simulink model "Optimisation01"  (R2020b)
settings: Solver=FixedStepAuto  StartTime=0.0  StopTime=10  FixedStep=0.01  MaxStep=0.2  RelTol=1e-3
model workspace (MAT data in the model file):
  Optimisation01_sdosession = sldodialogs.data.SessionData
  Optimisation01_sdosession.Version = '3.0'
  Optimisation01_sdosession.Data.ModelName = 'Optimisation01'
  Optimisation01_sdosession.Data.ToolType = 'ResponseOptimization'
  Optimisation01_sdosession.Data.GUIOptions.NoPromptClose = 0
  Optimisation01_sdosession.Data.Workspace.LocalWorkspace.DesignVars(1) = param.Continuous
  Optimisation01_sdosession.Data.Workspace.LocalWorkspace.DesignVars(1).Scale_ = 128
  Optimisation01_sdosession.Data.Workspace.LocalWorkspace.DesignVars(1).Size_ = [1 1]
  Optimisation01_sdosession.Data.Workspace.LocalWorkspace.DesignVars(1).Value_ = 50.1084192258
  Optimisation01_sdosession.Data.Workspace.LocalWorkspace.DesignVars(1).pID = paramid.Variable
  Optimisation01_sdosession.Data.Workspace.LocalWorkspace.DesignVars(1).pID.Name = 'Kd'
  Optimisation01_sdosession.Data.Workspace.LocalWorkspace.DesignVars(2) = param.Continuous
  Optimisation01_sdosession.Data.Workspace.LocalWorkspace.DesignVars(2).Scale_ = 8
  Optimisation01_sdosession.Data.Workspace.LocalWorkspace.DesignVars(2).Size_ = [1 1]
  Optimisation01_sdosession.Data.Workspace.LocalWorkspace.DesignVars(2).Value_ = 6.29568850936
  Optimisation01_sdosession.Data.Workspace.LocalWorkspace.DesignVars(2).pID = paramid.Variable
  Optimisation01_sdosession.Data.Workspace.LocalWorkspace.DesignVars(2).pID.Name = 'Ki'
  Optimisation01_sdosession.Data.Workspace.LocalWorkspace.DesignVars(3) = param.Continuous
  Optimisation01_sdosession.Data.Workspace.LocalWorkspace.DesignVars(3).Scale_ = 512
  Optimisation01_sdosession.Data.Workspace.LocalWorkspace.DesignVars(3).Size_ = [1 1]
  Optimisation01_sdosession.Data.Workspace.LocalWorkspace.DesignVars(3).Value_ = 364.260452278
  Optimisation01_sdosession.Data.Workspace.LocalWorkspace.DesignVars(3).pID = paramid.Variable
  Optimisation01_sdosession.Data.Workspace.LocalWorkspace.DesignVars(3).pID.Name = 'Kp'
  Optimisation01_sdosession.Data.Workspace.LocalWorkspace.ReqValues.Name = 'SignalProperty'
  Optimisation01_sdosession.Data.Workspace.LocalWorkspace.ReqValues.Type = 'min'
  Optimisation01_sdosession.Data.Workspace.LocalWorkspace.ReqValues.Value = 0.138601422932
  Optimisation01_sdosession.Data.Workspace.LocalWorkspace.ReqValues.DisplayValue = 0.138601422932
  Optimisation01_sdosession.Data.Workspace.LocalWorkspace.ReqValues_1.Name = 'SignalProperty'
  Optimisation01_sdosession.Data.Workspace.LocalWorkspace.ReqValues_1.Type = 'min'
  Optimisation01_sdosession.Data.Workspace.LocalWorkspace.ReqValues_1.Value = 0.264162161638
  Optimisation01_sdosession.Data.Workspace.LocalWorkspace.ReqValues_1.DisplayValue = 0.264162161638
  Optimisation01_sdosession.Data.Workspace.LocalWorkspace.Sig = Simulink.SimulationData.Signal
  Optimisation01_sdosession.Data.Workspace.LocalWorkspace.Sig.PortType = 'outport'
  Optimisation01_sdosession.Data.Workspace.LocalWorkspace.Sig.Version = 1
  Optimisation01_sdosession.Data.Workspace.LocalWorkspace.Sig.BlockPath = Simulink.SimulationData.BlockPath
  Optimisation01_sdosession.Data.Workspace.LocalWorkspace.Sig.BlockPath.path = {'Optimisation01/Sqrt'}
  Optimisation01_sdosession.Data.Workspace.LocalWorkspace.SignalProperty = sdo.requirements.SignalProperty
  Optimisation01_sdosession.Data.Workspace.LocalWorkspace.SignalProperty.sdo.requirements.Requirement.Data_ : srorequirement.functiondata (value not decoded)
  Optimisation01_sdosession.Data.Workspace.LocalWorkspace.SignalProperty.sdo.requirements.Requirement.Check_ = sdo.requirements.ScalarCheck
  Optimisation01_sdosession.Data.Workspace.HiddenWorkspace = []
  Optimisation01_sdosession.Data.ToolData.PlotManager.Plots(1).Class = 'sldoplots.TimePlot'
  Optimisation01_sdosession.Data.ToolData.PlotManager.Plots(1).Sources = {'Sig'}
  Optimisation01_sdosession.Data.ToolData.PlotManager.Plots(2).Class = 'sldoplots.IterPlot'
  Optimisation01_sdosession.Data.ToolData.PlotManager.Plots(2).Sources = {'SignalProperty'}
  Optimisation01_sdosession.Data.ToolData.PlotManager.Tiling : java.lang.String (value not decoded)
  Optimisation01_sdosession.Data.ToolData.DialogManager = []
  Optimisation01_sdosession.Data.ToolData.ResponseOptimization.Options = sdo.OptimizeOptions
  Optimisation01_sdosession.Data.ToolData.ResponseOptimization.Options.OptimizedModel = 'Optimisation01'
  Optimisation01_sdosession.Data.ToolData.ResponseOptimization.Options.Version = 2
  Optimisation01_sdosession.Data.ToolData.ResponseOptimization.GUIOptions.ModelTimeOut = Inf
  Optimisation01_sdosession.Data.ToolData.ResponseOptimization.GUIOptions.ComputeOperatingPoint = 0
  Optimisation01_sdosession.Data.ToolData.ResponseOptimization.GUIOptions.ShowProgress = 1
  Optimisation01_sdosession.Data.ToolData.ResponseOptimization.GUIOptions.ShowParamTrajectory = 1
  Optimisation01_sdosession.Data.ToolData.ResponseOptimization.GUIOptions.UpdatePlots = 1
  Optimisation01_sdosession.Data.ToolData.ResponseOptimization.GUIOptions.UpdateModel = 1
  Optimisation01_sdosession.Data.ToolData.ResponseOptimization.GUIOptions.UpdateDesign = 'overwrite'
  Optimisation01_sdosession.Data.ToolData.ResponseOptimization.GUIOptions.SaveReport = 0
  Optimisation01_sdosession.Data.ToolData.ResponseOptimization.GUIOptions.SaveRequirementValue = 1
  Optimisation01_sdosession.Data.ToolData.ResponseOptimization.LinOptions = linearize.LinearizeOptions
  Optimisation01_sdosession.Data.ToolData.ResponseOptimization.RequirementOperatingPointSetup = []
  Optimisation01_sdosession.Data.ToolData.ResponseOptimization.LocalRequirements.Requirement = 'SignalProperty'
  Optimisation01_sdosession.Data.ToolData.ResponseOptimization.LocalRequirements.Source = {'Sig'}
  Optimisation01_sdosession.Data.ToolData.ResponseOptimization.LocalRequirements.Selected = 1
  Optimisation01_sdosession.Data.ToolData.ResponseOptimization.BlockRequirements = struct([])
  Optimisation01_sdosession.Data.ToolData.ResponseOptimization.LocalExperiments = struct([])
  Optimisation01_sdosession.Data.ToolData.ResponseOptimization.Cost.Type = 'SSE'
  Optimisation01_sdosession.Data.ToolData.ResponseOptimization.Cost.Robust = 'off'
  Optimisation01_sdosession.Data.ToolData.ResponseOptimization.DesignVariables = 'DesignVars'
  Optimisation01_sdosession.Data.ToolData.ResponseOptimization.UncertainVariables = ''
  Optimisation01_sdosession.Data.ToolData.ResponseOptimization.DataToPlot = 'Sig'
values from neighbouring files (symbols this model uses):
  Kd = 138.349198174    [OptimisationData.mat]    (also in myCustomRequirement.m = data.DesignVars(3))
  Ki = 3.37771766611    [OptimisationData.mat]    (also in myCustomRequirement.m = data.DesignVars(2))
  Kp = 1303.85880325    [OptimisationData.mat]    (also in myCustomRequirement.m = data.DesignVars(1))
  Power = [0 0.135039524161 8.91914965689 7.78138466797 9.0073673393 8.96604203154 8.86759000228 15.68308669 17.9316117445 18.8693109472 25.7680840998 34.2690025221 ... (50 elements, 50x1)]    [MotorData.mat]    (also in OptimisationData.mat = [0 0.134792669981 8.9180951627 7.77881648635 9.00749423422 8)
  Throttle = [0 1 2.66666666667 3.44444444444 6.55555555556 8.11111111111 8.88888888889 13.6666666667 14.4444444444 15.2222222222 18.3333333333 21.5555555556 ... (50 elements, 50x1)]    [MotorData.mat]    (also in OptimisationData.mat)
  Thrust = [0 0.00386703849483 0.447248955951 0.381725752671 0.429816366755 0.448130327307 0.434268732353 0.786362880096 0.850043356053 0.907127881895 1.24377109743 1.5194958901 ... (50 elements, 50x1)]    [MotorData.mat]    (also in OptimisationData.mat)
libraries: simulink x2, pid_lib x1
settings Model: Creator=IR13  LastModifiedBy=IR13
settings SolverCC: ZeroCrossAlgorithm=Adaptive
settings DataIOCC: Refine=2
settings OptimizationCC: DefaultUnderspecifiedDataType=single
settings DebuggingCC: IgnoredZcDiagnostic=none

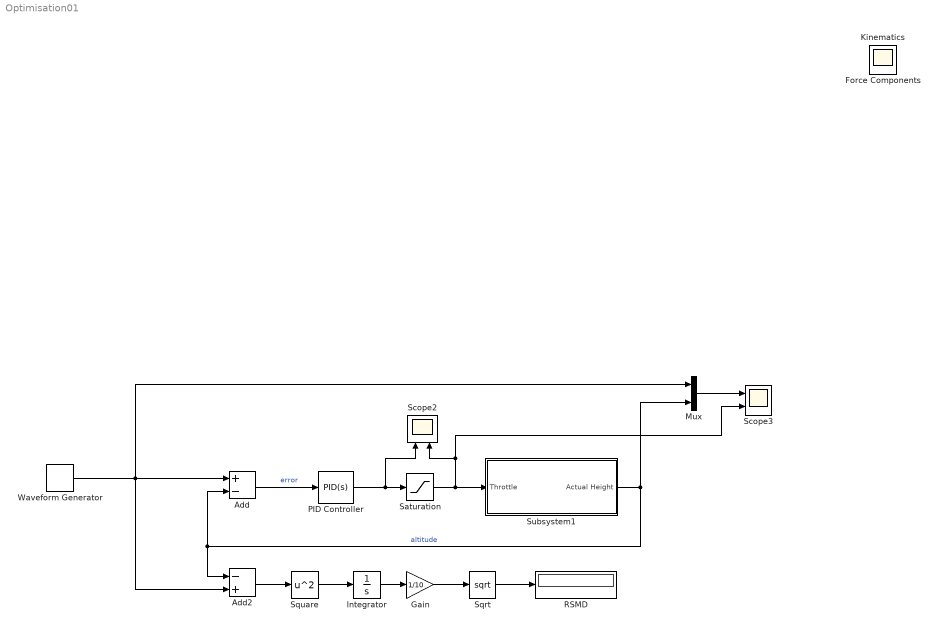
== system Optimisation01 ==
  Add : Sum  Inputs=+-
  Add2 : Sum  Inputs=-+
  Gain : Gain  Gain=1/10
  Integrator : Integrator
  Mux : Mux  Inputs=2
  PID Controller : pid_lib/PID Controller  Controller=PID  Form=Parallel  TimeDomain=Continuous-time  UseExternalTs=off  SampleTime=-1  IntegratorMethod=Forward Euler  FilterMethod=Forward Euler  ControllerParametersSource=internal  P=Kp  I=Ki  D=Kd  UseFilter=on  N=100  TunerSelectOption=Transfer Function Based (PID Tuner App)  InitialConditionSource=internal  InitialConditionForIntegrator=0  InitialConditionForFilter=0  DifferentiatorICPrevScaledInput=0  ExternalReset=none  TrackingMode=off  Kt=1  LimitOutput=off  SatLimitsSource=internal  UpperSaturationLimit=inf  LowerSaturationLimit=-inf  LinearizeAsGain=on  AntiWindupMode=none  Kb=1  POutMin=[]  POutMax=[]  IOutMin=[]  IOutMax=[]  DOutMin=[]  DOutMax=[]  NOutMin=[]  NOutMax=[]  SumOutMin=[]  SumOutMax=[]  SaturationOutMin=[]  SaturationOutMax=[]  PParamMin=[]  PParamMax=[]  IParamMin=[]  IParamMax=[]  DParamMin=[]  DParamMax=[]  NParamMin=[]  NParamMax=[]  KbParamMin=[]  KbParamMax=[]  KtParamMin=[]  KtParamMax=[]  KbOutMin=[]  KbOutMax=[]  KtOutMin=[]  KtOutMax=[]  IntegratorOutMin=[]  IntegratorOutMax=[]  FilterOutMin=[]  FilterOutMax=[]  SumI1OutMin=[]  SumI1OutMax=[]  SumI2OutMin=[]  SumI2OutMax=[]  SumI3OutMin=[]  SumI3OutMax=[]  SumI4OutMin=[]  SumI4OutMax=[]  SumDOutMin=[]  SumDOutMax=[]  DifferentiatorOutMin=[]  DifferentiatorOutMax=[]  FilterDiffOutCoefMin=[]  FilterDiffOutCoefMax=[]  ReciprocalOutMin=[]  ReciprocalOutMax=[]  SumDenOutMin=[]  SumDenOutMax=[]  SumNumOutMin=[]  SumNumOutMax=[]  DivideOutMin=[]  DivideOutMax=[]  UdiffTsProdOutMin=[]  UdiffTsProdOutMax=[]  NTsProdOutMin=[]  NTsProdOutMax=[]  UintegralTsProdOutMin=[]  UintegralTsProdOutMax=[]  UngainTsProdOutMin=[]  UngainTsProdOutMax=[]  IntegratorContinuousStateAttributes=''  IntegratorStateMustResolveToSignalObject=off  IntegratorRTWStateStorageClass=Auto  FilterContinuousStateAttributes=''  FilterStateMustResolveToSignalObject=off  FilterRTWStateStorageClass=Auto  ParallelPVariant=InternalParameters  IdealPVariant=Disabled  IVariant=InternalParameters  DVariant=InternalParameters  IntegratorVariant=Continuous  SatVariant=Disabled  AWVariant=Passthrough  PCopyVariant=Disabled  TRVariant=Disabled  FdbkBlocksVariant=Forward  IdealPFdbkVariant=Disabled  SatFdbkVariant=Disabled  DerivativeFilterVariant=ContFilter  NVariant=InternalParameters  NCopyVariant=Disabled  FilterICVariant=InternalICsFilter  IntegratorICVariant=InternalICs  ExternalResetVariant=Disabled  TRSumVariant=Passthrough  SumFdbkVariant=Disabled  SumVariant=Sum_PID  TsampFilterVariant=InternalTs  TsampNgainVariant=Passthrough  TsampIntegralVariant=Passthrough  ExternalSaturationOutDataTypeStr=Inherit: Same as second input
  RSMD : Display
  Saturation : Saturate  UpperLimit=100  LowerLimit=0
  Scope2 : Scope  NumInputPorts=2
  Scope3 : Scope  NumInputPorts=2
  Sqrt : Sqrt  SaturateOnIntegerOverflow=on
  Square : Math  Operator=square  SaturateOnIntegerOverflow=on
  Subsystem1 : Subsystem
  Waveform Generator : simulink/Sources/Waveform Generator  OutMin=[]  OutMax=[]  OutDataTypeStr=double  SelectedSignal=1  Signals=pulse(0.5, 2, 2) + pulse(1,5,2) + pulse(0.5,6,2)#pulse(1,4,2)#pulse(0.5,6,2)  BlockNames=MultiportSwitch_1f4ce5d91b3e4fe#MultiportSwitch_6a89107336d5467#MultiportSwitch_35f949fc017b494  SampleTime=0.1
  Force Components : Scope
  Kinematics : Scope
  wires:
  Saturation/1 -> Scope3/2, Scope2/2, Subsystem1/1(Throttle)
  Add2/1 -> Square/1
  Gain/1 -> Sqrt/1
  Add/1 -> PID Controller/1  "error"
  Waveform Generator/1 -> Mux/1, Add/1, Add2/2
  Square/1 -> Integrator/1
  Subsystem1/1(Actual Height) -> Mux/2, Add2/1, Add/2  "altitude"
  Sqrt/1 -> RSMD/1
  PID Controller/1 -> Scope2/1, Saturation/1
  Integrator/1 -> Gain/1
  Mux/1 -> Scope3/1

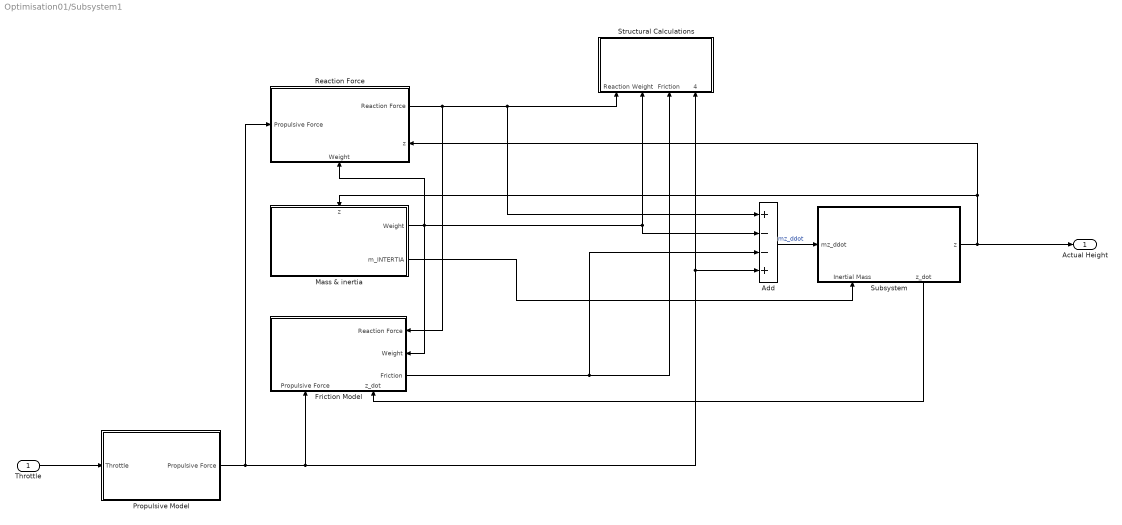
== system Optimisation01/Subsystem1 ==
  Throttle : Inport
  Add : Sum  Inputs=+--+
  Friction Model : Subsystem
      settings: PortSchema="{\"entries\":[{\"content\":{\"sides\":[{\"content\":{\"connectorIds\":[]},\"type\":\"ConnectorPlacement.EquallySpacedRectSide\",\"uuid\":\"1b3e095a-62ff-489c-96d9-63a8a1a842c7\"},{\"content\":{\"connectorIds\":[\"In3\",\"In4\",\"Out1\"],\"side\":\"RIGHT\"},\"type\":\"ConnectorPlacement.EquallySpacedRectSide\",\"uuid\":\"2aa3988f-f37b-48ca-a763-ece382c29199\"},{\"content\":{\"connectorIds\":[],\"side\":\"TOP\"},\"type\":\"ConnectorPlacement.EquallySpacedRectSide\",\"uuid\":\"ef7ffbd1-84d2-4291-ae41-90f24840b975\"},{\"content\":{\"connectorIds\":[\"In1\",\"In2\"],\"side\":\"BOTTOM\"},\"type\":\"ConnectorPlacement.EquallySpacedRectSide\",\"uuid\":\"ca187e87-455c-44d4-b2d5-496c3fe29e76\"},{\"content\":{\"connectorIds\":[],\"side\":\"HIDDEN\"},\"type\":\"ConnectorPlacement.EquallySpacedRectSide\",\"uuid\":\"11859c76-ab54-4977-b256-12d02241e5aa\"}]},\"type\":\"ConnectorPlacement.EquallySpacedConnector\",\"uuid\":\"162037a6-f725-4d16-a5f0-9112b8e8c48a\"}],\"packageUris\":[\"http://schema.mathworks.com/mf0/Connector/R2020b\"],\"version\":\"1.0\"}"
  Mass & inertia : Subsystem
      settings: PortSchema="{\"entries\":[{\"content\":{\"sides\":[{\"content\":{\"connectorIds\":[]},\"type\":\"ConnectorPlacement.EquallySpacedRectSide\",\"uuid\":\"1399d11e-8fed-4a75-a6ac-2b525e4dbe81\"},{\"content\":{\"connectorIds\":[\"Out1\",\"Out2\"],\"side\":\"RIGHT\"},\"type\":\"ConnectorPlacement.EquallySpacedRectSide\",\"uuid\":\"2e2e7a23-dcb2-4001-96a5-c1562d5723c6\"},{\"content\":{\"connectorIds\":[\"In1\"],\"side\":\"TOP\"},\"type\":\"ConnectorPlacement.EquallySpacedRectSide\",\"uuid\":\"b0373260-5e1a-43dd-bca8-24421c20e285\"},{\"content\":{\"connectorIds\":[],\"side\":\"HIDDEN\"},\"type\":\"ConnectorPlacement.EquallySpacedRectSide\",\"uuid\":\"35e9db29-fffd-4860-9f0e-8f51711f4d01\"}]},\"type\":\"ConnectorPlacement.EquallySpacedConnector\",\"uuid\":\"39bd9006-0e99-41e8-8a89-05408a55c646\"}],\"packageUris\":[\"http://schema.mathworks.com/mf0/Connector/R2020b\"],\"version\":\"1.0\"}"
  Propulsive Model : Subsystem
  Reaction Force : Subsystem
      settings: PortSchema="{\"entries\":[{\"content\":{\"sides\":[{\"content\":{\"connectorIds\":[\"In1\"]},\"type\":\"ConnectorPlacement.EquallySpacedRectSide\",\"uuid\":\"1e35d603-08eb-402b-a2de-16d799202cf1\"},{\"content\":{\"connectorIds\":[\"Out1\",\"In3\"],\"side\":\"RIGHT\"},\"type\":\"ConnectorPlacement.EquallySpacedRectSide\",\"uuid\":\"6309f8f8-5c50-477a-b178-9a414ecebc78\"},{\"content\":{\"connectorIds\":[],\"side\":\"TOP\"},\"type\":\"ConnectorPlacement.EquallySpacedRectSide\",\"uuid\":\"1075b443-bbcc-4bf5-9b05-7b44ecc9bacc\"},{\"content\":{\"connectorIds\":[\"In2\"],\"side\":\"BOTTOM\"},\"type\":\"ConnectorPlacement.EquallySpacedRectSide\",\"uuid\":\"9465d0d7-9803-4a37-84cd-7fa866de481e\"},{\"content\":{\"connectorIds\":[],\"side\":\"HIDDEN\"},\"type\":\"ConnectorPlacement.EquallySpacedRectSide\",\"uuid\":\"80b90c9b-51c1-4183-87d9-243ed5e6c391\"}]},\"type\":\"ConnectorPlacement.EquallySpacedConnector\",\"uuid\":\"514452d4-5b8b-4aa9-8f6a-f7d3b564ce33\"}],\"packageUris\":[\"http://schema.mathworks.com/mf0/Connector/R2020b\"],\"version\":\"1.0\"}"
  Structural Calculations : Subsystem
  Subsystem : Subsystem
      settings: PortSchema="{\"entries\":[{\"content\":{\"sides\":[{\"content\":{\"connectorIds\":[\"In1\"]},\"type\":\"ConnectorPlacement.EquallySpacedRectSide\",\"uuid\":\"4280b032-842d-4d16-b8c5-b63b72592cbb\"},{\"content\":{\"connectorIds\":[\"Out1\"],\"side\":\"RIGHT\"},\"type\":\"ConnectorPlacement.EquallySpacedRectSide\",\"uuid\":\"e4e0b7b9-12b8-4ae8-8e3c-cb8798002b22\"},{\"content\":{\"connectorIds\":[],\"side\":\"TOP\"},\"type\":\"ConnectorPlacement.EquallySpacedRectSide\",\"uuid\":\"d9ed1db6-3da5-4dd5-916f-0a0888e518e7\"},{\"content\":{\"connectorIds\":[\"In2\",\"Out2\"],\"side\":\"BOTTOM\"},\"type\":\"ConnectorPlacement.EquallySpacedRectSide\",\"uuid\":\"d18e58c7-4d86-4b90-a916-d0a361083c2d\"},{\"content\":{\"connectorIds\":[],\"side\":\"HIDDEN\"},\"type\":\"ConnectorPlacement.EquallySpacedRectSide\",\"uuid\":\"56aebb37-ad12-4a95-93b1-0a5b21e6f2e4\"}]},\"type\":\"ConnectorPlacement.EquallySpacedConnector\",\"uuid\":\"f0e8b7a0-91bd-4506-81db-435517f4e301\"}],\"packageUris\":[\"http://schema.mathworks.com/mf0/Connector/R2020b\"],\"version\":\"1.0\"}"
  Actual Height : Outport
  wires:
  Reaction Force/1(Reaction Force) -> Add/1, Structural Calculations/1(Reaction), Friction Model/3(Reaction Force)
  Mass & inertia/2(m_INTERTIA) -> Subsystem/2(Inertial Mass)
  Throttle/1 -> Propulsive Model/1(Throttle)
  Subsystem/1(z) -> Actual Height/1, Reaction Force/3(z), Mass & inertia/1(z)
  Subsystem/2(z_dot) -> Friction Model/2(z_dot)
  Propulsive Model/1(Propulsive Force) -> Add/4, Structural Calculations/4(Propulsion), Friction Model/1(Propulsive Force), Reaction Force/1(Propulsive Force)
  Add/1 -> Subsystem/1(mz_ddot)  "mz_ddot"
  Mass & inertia/1(Weight) -> Friction Model/4(Weight), Reaction Force/2(Weight), Structural Calculations/2(Weight), Add/2
  Friction Model/1(Friction) -> Add/3, Structural Calculations/3(Friction)

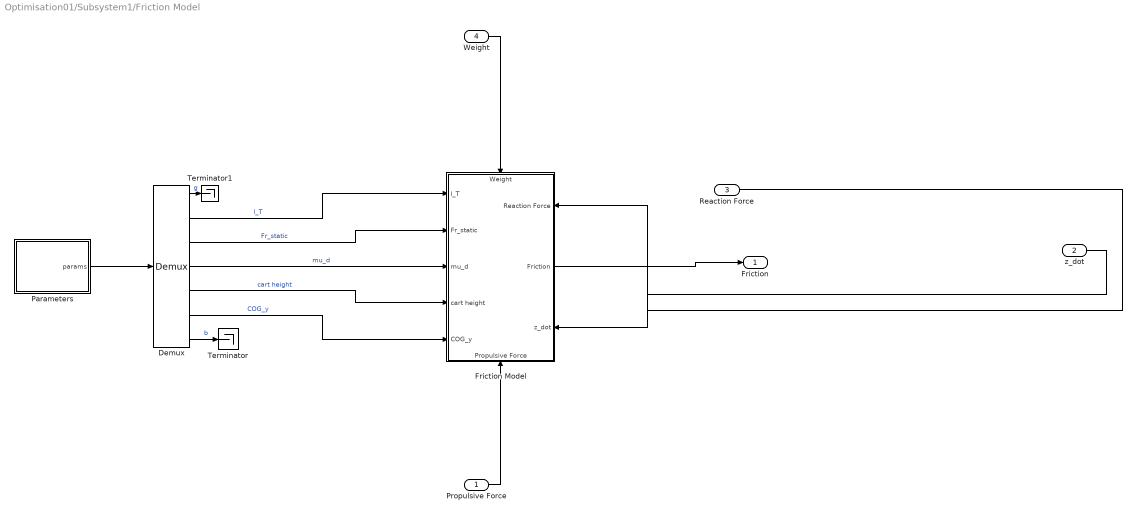
== system Optimisation01/Subsystem1/Friction Model ==
  Propulsive Force : Inport
  z_dot : Inport  Port=2
  Reaction Force : Inport  Port=3
  Weight : Inport  Port=4
  Demux : Demux  Outputs=7
  Friction Model : Subsystem
      settings: PortSchema="{\"entries\":[{\"content\":{\"sides\":[{\"content\":{\"connectorIds\":[\"In1\",\"In2\",\"In3\",\"In4\",\"In5\"]},\"type\":\"ConnectorPlacement.EquallySpacedRectSide\",\"uuid\":\"b80da770-fdb0-4d6f-bea5-94e06f2afa04\"},{\"content\":{\"connectorIds\":[\"In8\",\"Out1\",\"In9\"],\"side\":\"RIGHT\"},\"type\":\"ConnectorPlacement.EquallySpacedRectSide\",\"uuid\":\"44cc0c5b-7bc2-4d7d-ab9c-4e4237bff03f\"},{\"content\":{\"connectorIds\":[\"In6\"],\"side\":\"TOP\"},\"type\":\"ConnectorPlacement.EquallySpacedRectSide\",\"uuid\":\"d8cf9831-f5c9-4bfd-8650-bb94040859dc\"},{\"content\":{\"connectorIds\":[\"In7\"],\"side\":\"BOTTOM\"},\"type\":\"ConnectorPlacement.EquallySpacedRectSide\",\"uuid\":\"5dc8ad5a-b457-4b35-ae96-3ded03a76763\"},{\"content\":{\"connectorIds\":[],\"side\":\"HIDDEN\"},\"type\":\"ConnectorPlacement.EquallySpacedRectSide\",\"uuid\":\"8dab3da8-cd9e-407c-8850-bafd2d7a131e\"}]},\"type\":\"ConnectorPlacement.EquallySpacedConnector\",\"uuid\":\"d0f16782-5cb8-4cea-b1e1-f78879901c5f\"}],\"packageUris\":[\"http://schema.mathworks.com/mf0/Connector/R2020b\"],\"version\":\"1.0\"}"
  Parameters : MATLAB Function  TreatAsAtomicUnit=on
  Terminator : Terminator
  Terminator1 : Terminator
  Friction : Outport
  wires:
  Demux/7 -> Terminator/1  "b"
  Reaction Force/1 -> Friction Model/8(Reaction Force)
  Demux/1 -> Terminator1/1  "g"
  Propulsive Force/1 -> Friction Model/7(Propulsive Force)
  Demux/2 -> Friction Model/1(l_T)  "l_T"
  Friction Model/1(Friction) -> Friction/1
  Weight/1 -> Friction Model/6(Weight)
  Demux/3 -> Friction Model/2(Fr_static)  "Fr_static"
  Parameters/1(params) -> Demux/1
  Demux/4 -> Friction Model/3(mu_d)  "mu_d"
  z_dot/1 -> Friction Model/9(z_dot)
  Demux/5 -> Friction Model/4(cart height)  "cart height"
  Demux/6 -> Friction Model/5(COG_y)  "COG_y"

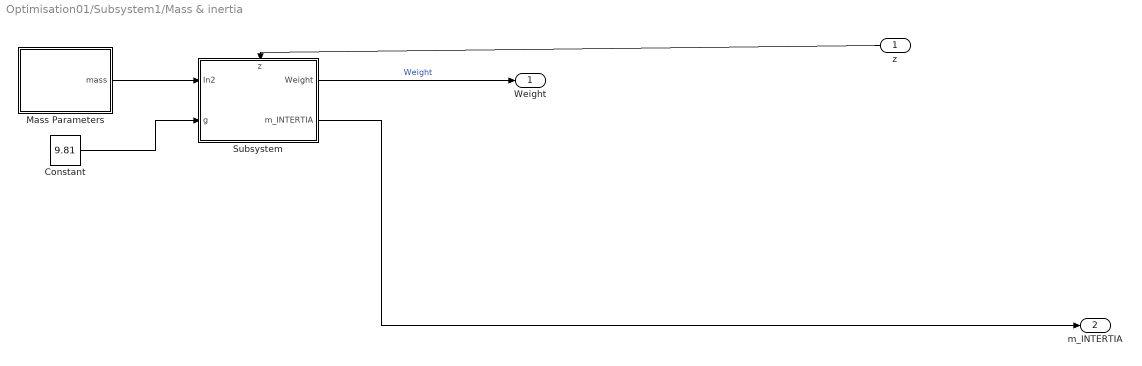
== system Optimisation01/Subsystem1/Mass & inertia ==
  z : Inport
  Constant : Constant  Value=9.81
  Mass Parameters : MATLAB Function  TreatAsAtomicUnit=on
  Subsystem : Subsystem
      settings: PortSchema="{\"entries\":[{\"content\":{\"sides\":[{\"content\":{\"connectorIds\":[\"In1\",\"In2\"]},\"type\":\"ConnectorPlacement.EquallySpacedRectSide\",\"uuid\":\"22ad1645-0c4a-4eab-a942-e35708909bc2\"},{\"content\":{\"connectorIds\":[\"Out1\",\"Out2\"],\"side\":\"RIGHT\"},\"type\":\"ConnectorPlacement.EquallySpacedRectSide\",\"uuid\":\"049dc02c-af21-4242-96fd-198a717a970b\"},{\"content\":{\"connectorIds\":[\"In3\"],\"side\":\"TOP\"},\"type\":\"ConnectorPlacement.EquallySpacedRectSide\",\"uuid\":\"a1727784-13c5-452f-b8c4-4da743b82409\"},{\"content\":{\"connectorIds\":[],\"side\":\"HIDDEN\"},\"type\":\"ConnectorPlacement.EquallySpacedRectSide\",\"uuid\":\"a08d060c-4763-496d-ac54-202c99d24543\"}]},\"type\":\"ConnectorPlacement.EquallySpacedConnector\",\"uuid\":\"dcd15304-2046-43f2-990d-e6438030fbb8\"}],\"packageUris\":[\"http://schema.mathworks.com/mf0/Connector/R2020b\"],\"version\":\"1.0\"}"
  Weight : Outport
  m_INTERTIA : Outport  Port=2
  wires:
  Subsystem/2(m_INTERTIA) -> m_INTERTIA/1
  Constant/1 -> Subsystem/2(g)
  Subsystem/1(Weight) -> Weight/1  "Weight"
  z/1 -> Subsystem/3(z)
  Mass Parameters/1(mass) -> Subsystem/1(In2)

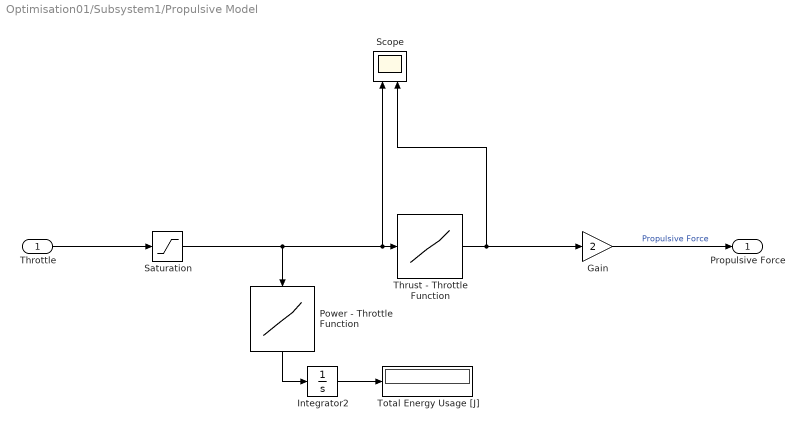
== system Optimisation01/Subsystem1/Propulsive Model ==
  Throttle : Inport
  Gain : Gain  Gain=2
  Integrator2 : Integrator
  Power - Throttle Function : Lookup_n-D  NumberOfTableDimensions=1  BreakpointsForDimension1=Throttle  BreakpointsForDimension2=[1:3]  Table=Power  ExtrapMethod=Clip  InternalRulePriority=Speed  RndMeth=Simplest  InputSameDT=on
  Saturation : Saturate  UpperLimit=100  LowerLimit=0
  Scope : Scope  NumInputPorts=2
  Thrust - Throttle Function : Lookup_n-D  NumberOfTableDimensions=1  BreakpointsForDimension1=Throttle  BreakpointsForDimension2=[1:3]  Table=Thrust  ExtrapMethod=Clip  DiagnosticForOutOfRangeInput=Warning  InternalRulePriority=Speed  RndMeth=Simplest  InputSameDT=on
  Total Energy Usage [J] : Display
  Propulsive Force : Outport
  wires:
  Integrator2/1 -> Total Energy Usage [J]/1
  Thrust - Throttle Function/1 -> Gain/1, Scope/2
  Power - Throttle Function/1 -> Integrator2/1
  Gain/1 -> Propulsive Force/1  "Propulsive Force"
  Throttle/1 -> Saturation/1
  Saturation/1 -> Scope/1, Thrust - Throttle Function/1, Power - Throttle Function/1

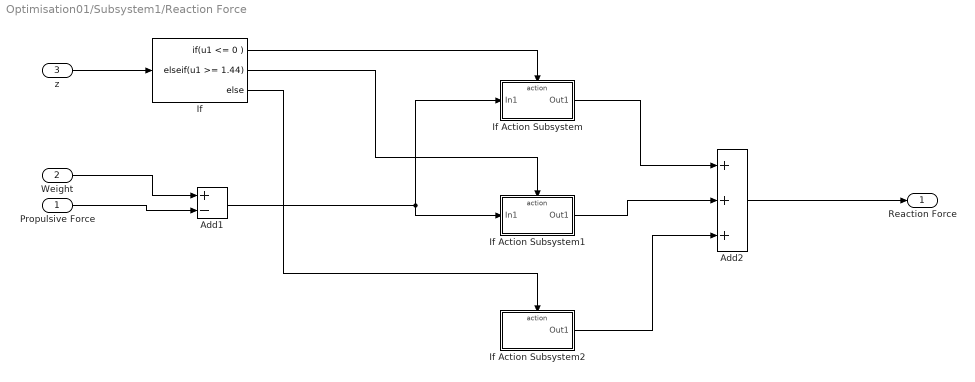
== system Optimisation01/Subsystem1/Reaction Force ==
  Propulsive Force : Inport
  Weight : Inport  Port=2
  z : Inport  Port=3
  Add1 : Sum  Inputs=+-
  Add2 : Sum  Inputs=+++
  If : If  IfExpression=u1 <= 0  ElseIfExpressions=u1 >= 1.44
  If Action Subsystem : Subsystem  TreatAsAtomicUnit=on
  If Action Subsystem1 : Subsystem  TreatAsAtomicUnit=on
  If Action Subsystem2 : Subsystem  TreatAsAtomicUnit=on
  Reaction Force : Outport
  wires:
  Weight/1 -> Add1/1
  If Action Subsystem1/1(Out1) -> Add2/2
  z/1 -> If/1
  Add2/1 -> Reaction Force/1
  If/2 -> If Action Subsystem1/Action
  If Action Subsystem2/1(Out1) -> Add2/3
  Propulsive Force/1 -> Add1/2
  If Action Subsystem/1(Out1) -> Add2/1
  If/3 -> If Action Subsystem2/Action
  If/1 -> If Action Subsystem/Action
  Add1/1 -> If Action Subsystem1/1(In1), If Action Subsystem/1(In1)

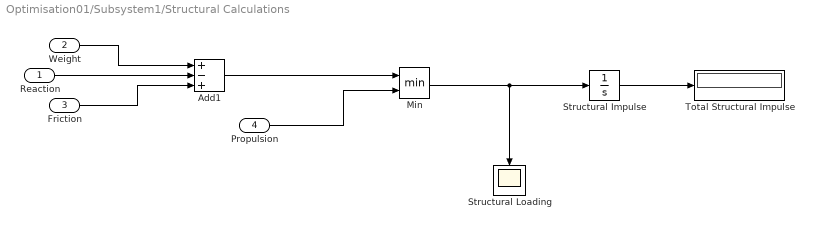
== system Optimisation01/Subsystem1/Structural Calculations ==
  Reaction : Inport
  Weight : Inport  Port=2
  Friction : Inport  Port=3
  Propulsion : Inport  Port=4
  Add1 : Sum  Inputs=+-+
  Min : MinMax  Inputs=2
  Structural Impulse : Integrator
  Structural Loading : Scope
  Total Structural Impulse : Display
  wires:
  Propulsion/1 -> Min/2
  Friction/1 -> Add1/3
  Min/1 -> Structural Loading/1, Structural Impulse/1
  Weight/1 -> Add1/1
  Reaction/1 -> Add1/2
  Structural Impulse/1 -> Total Structural Impulse/1
  Add1/1 -> Min/1

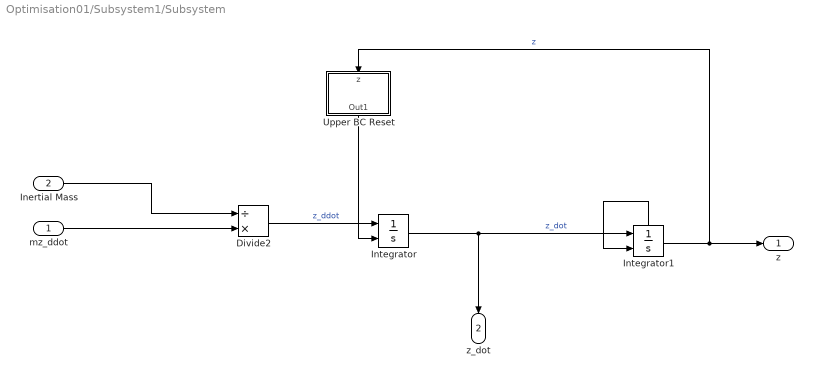
== system Optimisation01/Subsystem1/Subsystem ==
  mz_ddot : Inport
  Inertial Mass : Inport  Port=2
  Divide2 : Product  Inputs=/*
  Integrator : Integrator  ExternalReset=falling
  Integrator1 : Integrator  ExternalReset=falling  ShowStatePort=on
  Upper BC Reset : Subsystem
  z : Outport
  z_dot : Outport  Port=2
  wires:
  mz_ddot/1 -> Divide2/2
  Upper BC Reset/1(Out1) -> Integrator/2
  Inertial Mass/1 -> Divide2/1
  Divide2/1 -> Integrator/1  "z_ddot"
  Integrator1/State -> Integrator1/2
  Integrator1/1 -> Upper BC Reset/1(z), z/1  "z"
  Integrator/1 -> z_dot/1, Integrator1/1  "z_dot"

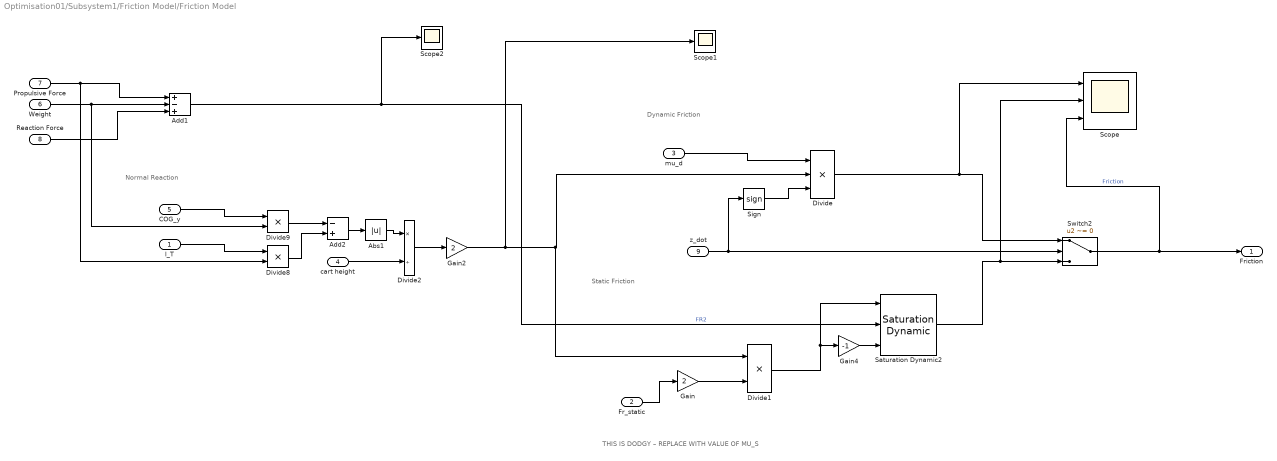
== system Optimisation01/Subsystem1/Friction Model/Friction Model ==
  note: Static Friction
  note: Dynamic Friction
  note: Normal Reaction
  note: THIS IS DODGY – REPLACE WITH VALUE OF MU_S
  l_T : Inport
  Fr_static : Inport  Port=2
  mu_d : Inport  Port=3
  cart height : Inport  Port=4
  COG_y : Inport  Port=5
  Weight : Inport  Port=6
  Propulsive Force : Inport  Port=7
  Reaction Force : Inport  Port=8
  z_dot : Inport  Port=9
  Abs1 : Abs
  Add1 : Sum  Inputs=+-+
  Add2 : Sum  Inputs=-+
  Divide : Product  Inputs=***
  Divide1 : Product  Inputs=**
  Divide2 : Product  Inputs=*/
  Divide8 : Product  Inputs=**
  Divide9 : Product  Inputs=**
  Gain : Gain  Gain=2
  Gain2 : Gain  Gain=2
  Gain4 : Gain  Gain=-1
  Saturation Dynamic2 : simulink/Discontinuities/Saturation Dynamic  OutMin=[]  OutMax=[]  OutDataTypeStr=Inherit: Same as second input  OutDataType=fixdt(1, 16)  OutScaling=2^-10  DoSatur=off
  Scope : Scope  NumInputPorts=3
  Scope1 : Scope
  Scope2 : Scope
  Sign : Signum
  Switch2 : Switch  Criteria=u2 ~= 0
  Friction : Outport
  wires:
  Reaction Force/1 -> Add1/3
  Add2/1 -> Abs1/1
  COG_y/1 -> Divide9/1
  cart height/1 -> Divide2/2
  Divide2/1 -> Gain2/1
  Divide9/1 -> Add2/1
  Divide8/1 -> Add2/2
  Weight/1 -> Add1/2, Divide9/2
  Abs1/1 -> Divide2/1
  Propulsive Force/1 -> Divide8/2, Add1/1
  l_T/1 -> Divide8/1
  Switch2/1 -> Scope/3, Friction/1  "Friction"
  Divide/1 -> Scope/1, Switch2/1
  mu_d/1 -> Divide/1
  Sign/1 -> Divide/3
  z_dot/1 -> Sign/1, Switch2/2
  Add1/1 -> Scope2/1, Saturation Dynamic2/2  "FR2"
  Saturation Dynamic2/1 -> Scope/2, Switch2/3
  Divide1/1 -> Saturation Dynamic2/1, Gain4/1
  Gain4/1 -> Saturation Dynamic2/3
  Fr_static/1 -> Gain/1
  Gain/1 -> Divide1/2
  Gain2/1 -> Scope1/1, Divide1/1, Divide/2

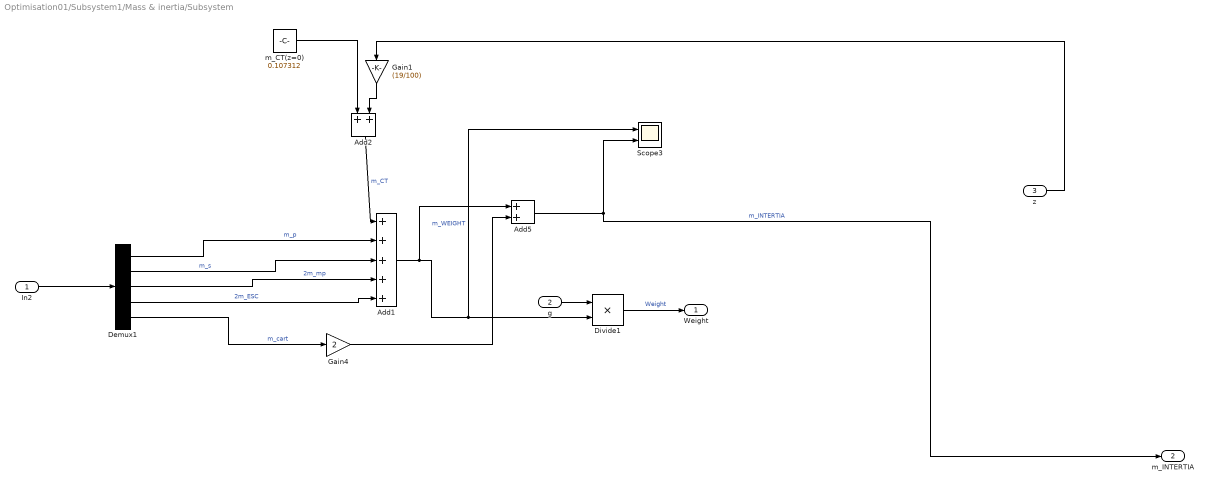
== system Optimisation01/Subsystem1/Mass & inertia/Subsystem ==
  In2 : Inport
  g : Inport  Port=2
  z : Inport  Port=3
  Add1 : Sum  Inputs=+++++
  Add2 : Sum
  Add5 : Sum
  Demux1 : Demux  Outputs=5
  Divide1 : Product  Inputs=**
  Gain1 : Gain  Gain=(19/100)
  Gain4 : Gain  Gain=2
  Scope3 : Scope  NumInputPorts=2
  m_CT(z=0) : Constant  Value=0.107312
  Weight : Outport
  m_INTERTIA : Outport  Port=2
  wires:
  Demux1/5 -> Gain4/1  "m_cart"
  Demux1/2 -> Add1/3  "m_s"
  Demux1/1 -> Add1/2  "m_p"
  Divide1/1 -> Weight/1  "Weight"
  Add2/1 -> Add1/1  "m_CT"
  In2/1 -> Demux1/1
  Gain4/1 -> Add5/2
  g/1 -> Divide1/1
  Gain1/1 -> Add2/2
  Add5/1 -> m_INTERTIA/1, Scope3/2  "m_INTERTIA"
  z/1 -> Gain1/1
  m_CT(z=0)/1 -> Add2/1
  Demux1/3 -> Add1/4  "2m_mp"
  Demux1/4 -> Add1/5  "2m_ESC"
  Add1/1 -> Add5/1, Scope3/1, Divide1/2  "m_WEIGHT"

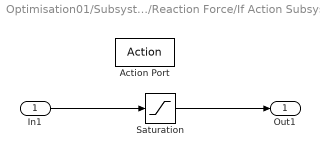
== system Optimisation01/Subsystem1/Reaction Force/If Action Subsystem ==
  In1 : Inport
  Action Port : ActionPort  ActionPortLabel=if(u1 <= 0 )
  Saturation : Saturate  UpperLimit=+inf  LowerLimit=0
  Out1 : Outport
  wires:
  In1/1 -> Saturation/1
  Saturation/1 -> Out1/1

== system Optimisation01/Subsystem1/Reaction Force/If Action Subsystem1 ==
  In1 : Inport
  Action Port : ActionPort  ActionPortLabel=elseif(u1 >= 1.44)
  Saturation : Saturate  UpperLimit=0  LowerLimit=-inf
  Out1 : Outport
  wires:
  In1/1 -> Saturation/1
  Saturation/1 -> Out1/1

== system Optimisation01/Subsystem1/Reaction Force/If Action Subsystem2 ==
  Action Port : ActionPort  ActionPortLabel=else
  Constant : Constant  Value=0
  Out1 : Outport
  wires:
  Constant/1 -> Out1/1

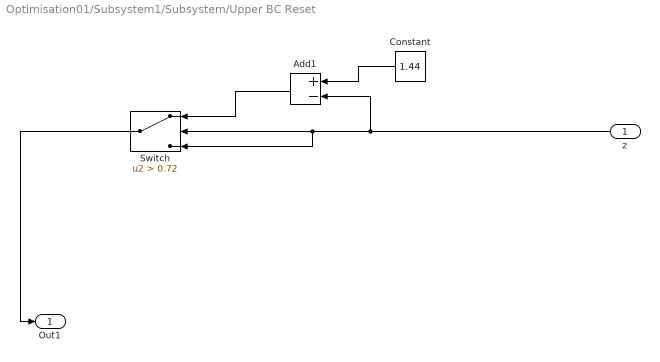
== system Optimisation01/Subsystem1/Subsystem/Upper BC Reset ==
  z : Inport
  Add1 : Sum  Inputs=+-
  Constant : Constant  Value=1.44
  Switch : Switch  Criteria=u2 > Threshold  Threshold=0.72
  Out1 : Outport
  wires:
  Add1/1 -> Switch/1
  Switch/1 -> Out1/1
  z/1 -> Add1/2, Switch/3, Switch/2
  Constant/1 -> Add1/1

== matlab function Optimisation01/Subsystem1/Friction Model/Parameters ==
  data: params output
function params = fcn()

%raw parameters
g = 9.81;
lT = 10; %y position of thrust point [mm]
F_r_static = 0.13; %static friction force [kgf]
mu_d = 0.14; %dynamic friction coefficient 
cart_height = 210.4; %[mm]
CoG_y = 10; %%[mm]
b = 0.2; %damping constant

params = [g;lT;F_r_static; mu_d; cart_height;CoG_y;b];

== matlab function Optimisation01/Subsystem1/Mass & inertia/Mass Parameters ==
  data: mass output
function mass = fcn()

%raw parameters

m_p = 0.15;
m_s = 0.2;
m_mp = 0.202; %mass of one motor prop
m_ESC = 0.102;
m_cart = 0.4; %mass of one cart without additional stuff


mass = [m_p;m_s;m_mp;m_ESC;m_cart];
